simulink model "kinctrlkinova"  (Simulink 8.9)
settings: Solver=ode45  StartTime=0.0  StopTime=20.0  MaxStep=0.1  RelTol=1e-5  EnableMultiTasking=on
values from neighbouring files (symbols this model uses):
  K = 1    [ex3.m]    (also in mdl_kinovagen3.m = 8.91)
  qr = [0 0  0 90 180 0 0]*pi/180    [mdl_kinovagen3.m]    (also in planar3dof.m = [0 pi/2 -pi])
libraries: roblocks x4, simulink x2
settings Model: LogicAnalyzerSignalOrdering=64fa8478-15b0-4dc5-9603-efdfb24b41bc  SuppressorTable=22 serialization::archive 11 0 6 0 0 0 11 0  Creator=fernando  LastModifiedBy=rbp
settings DataIOCC: SignalLoggingSaveFormat=Dataset
settings OptimizationCC: ExpressionDepthLimit=2147483647
settings DebuggingCC: SolverPrmCheckMsg=warning  AllowSymbolicDim=off

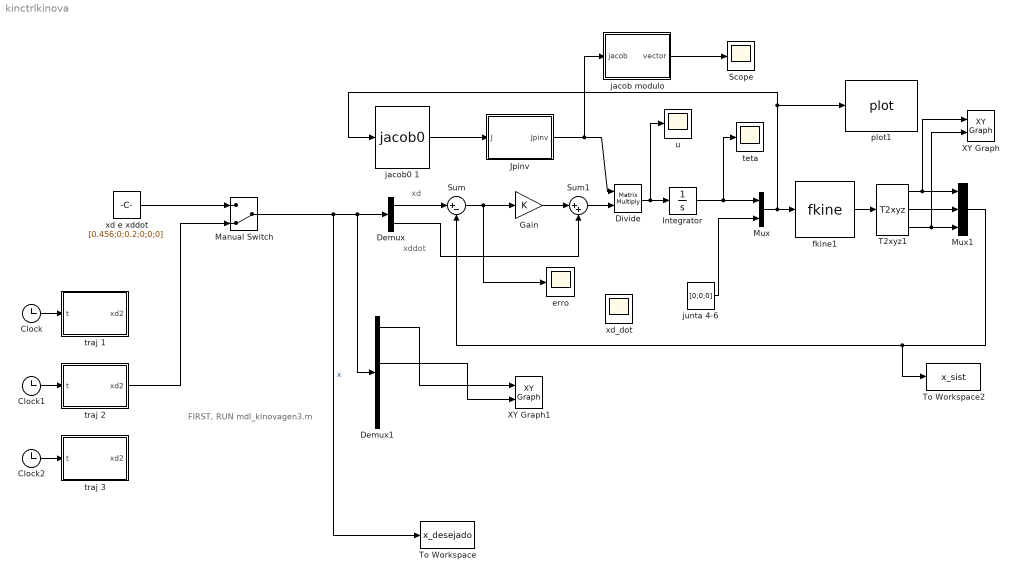
== system kinctrlkinova ==
  note: xd
  note: xddot
  note: FIRST, RUN mdl_kinovagen3.m
  Clock : Clock
  Clock1 : Clock
  Clock2 : Clock
  Demux : Demux  Outputs=2
  Demux1 : Demux  Outputs=6
  Divide : Product  Inputs=**  Multiplication=Matrix(*)
  Gain : Gain  Gain=K
  Integrator : Integrator  InitialCondition=qr(1:4)
  Jpinv : MATLAB Function  TreatAsAtomicUnit=on
  Manual Switch : ManualSwitch  CurrentSetting=0
  Mux : Mux  Inputs=2
  Mux1 : Mux  Inputs=3
  Scope : Scope
  Sum : Sum  Inputs=|+-
  Sum1 : Sum  Inputs=|++
  T2xyz1 : roblocks/Toolbox/T2xyz
  To Workspace : ToWorkspace  VariableName=x_desejado  SaveFormat=Timeseries  SampleTime=-1
  To Workspace2 : ToWorkspace  VariableName=x_sist  SaveFormat=Structure With Time  SampleTime=-1
  XY Graph : simulink/Sinks/XY Graph  xmin=-0  xmax=0.8  ymin=-0.3  ymax=0.5  st=-1
  XY Graph1 : simulink/Sinks/XY Graph  xmin=-0  xmax=0.8  ymin=-0.3  ymax=0.5  st=-1
  erro : Scope
  fkine1 : roblocks/Arm/fkine  robot=gen3
  jacob modulo : MATLAB Function  TreatAsAtomicUnit=on
  jacob0 1 : roblocks/Arm/jacob0   robot=gen3
  junta 4-6 : Constant  Value=[0;0;0]
  plot1 : roblocks/Arm/plot  robot=gen3  fps=5  holdplot=on
  teta : Scope
  traj 1 : MATLAB Function  TreatAsAtomicUnit=on
  traj 2 : MATLAB Function  TreatAsAtomicUnit=on
  traj 3 : MATLAB Function  TreatAsAtomicUnit=on
  u : Scope
  xd e xddot : Constant  Value=[0.456;0;0.2;0;0;0]
  xd_dot : Scope
  wires:
  Mux/1 -> fkine1/1, jacob0 1/1, plot1/1
  Integrator/1 -> Mux/1, teta/1
  junta 4-6/1 -> Mux/2
  Divide/1 -> Integrator/1, u/1
  Jpinv/1(Jpinv) -> jacob modulo/1(jacob), Divide/1
  Sum/1 -> Gain/1, erro/1
  T2xyz1/1 -> Mux1/1, XY Graph/1
  T2xyz1/2 -> Mux1/2
  T2xyz1/3 -> Mux1/3, XY Graph/2
  Mux1/1 -> To Workspace2/1, Sum/2
  jacob0 1/1 -> Jpinv/1(J)
  xd e xddot/1 -> Manual Switch/1
  Clock/1 -> traj 1/1(t)
  Manual Switch/1 -> To Workspace/1, Demux1/1, Demux/1  "x"
  Demux/1 -> Sum/1
  Gain/1 -> Sum1/1
  Sum1/1 -> Divide/2
  fkine1/1 -> T2xyz1/1
  Demux1/1 -> XY Graph1/1
  Demux1/3 -> XY Graph1/2
  Clock1/1 -> traj 2/1(t)
  Clock2/1 -> traj 3/1(t)
  jacob modulo/1(vector) -> Scope/1
  Demux/2 -> Sum1/2
  traj 2/1(xd2) -> Manual Switch/2

== matlab function Jpinv ==
  data: J input double; Jpinv output double
function Jpinv = fcn(J)
%#codegen

Jpinv = pinv(J(1:3,1:4));

== matlab function traj 1 ==
  data: t input double; xd2 output double
function xd2  = fcn(t)
%#codegen

wn=2*pi/10;

x = 0.075 * (sin(wn * t) + sin(4 * wn * t)) + 0.456;
z = 0.075 * (cos(wn * t) + cos(4 * wn * t)) + 0.069;

x_ponto = 0.075 * wn * (cos(wn * t) + 4*cos(4 * wn * t));
z_ponto = -0.075 * wn * (sin(wn * t) + 4*sin(4 * wn * t));

xd= [x 0 z]';
xddot= [x_ponto 0 z_ponto]';

 
 
xd2=[xd;xddot];

== matlab function jacob modulo ==
  data: jacob input double; vector output double
function vector  = fcn(jacob)
%#codegen

M = norm(jacob); 
 
vector=M;

== matlab function traj 2 ==
  data: t input double; xd2 output double
function xd2  = fcn(t)
%#codegen

wn=2*pi/10;

x = 0.075 * sin(wn * t) + 0.456;
z = 0.075 * cos(wn * t) + 0.2;

x_ponto = 0.075 * wn * cos(wn * t);
z_ponto = -0.075 * wn * sin(wn * t);

xd= [x 0 z]';
xddot= [x_ponto 0 z_ponto]';

 
 
xd2=[xd;xddot];

== matlab function traj 3 ==
  data: t input double; xd2 output double
function xd2  = fcn(t)
%#codegen

wn=2*pi/10;

x = 0.075 * sin(wn * t) + 0.456;
z = 0.075 * cos(wn * t) + 0.2;
y = (x - 0.456) + (z - 0.2);

x_ponto = 0.075 * wn * cos(wn * t);
y_ponto = 0.075 * wn * (cos(wn * t) - sin(wn * t));
z_ponto = -0.075 * wn * sin(wn * t);

xd= [x y z]';
xddot= [x_ponto y_ponto z_ponto]';

 
 
xd2=[xd;xddot];
